simulink model "RoboBoatVU_2014_Athena"  (R2014a)
settings: Solver=FixedStepDiscrete  StartTime=0.0  StopTime=inf  FixedStep=.1  RelTol=1e-3
undefined symbols (not defined in the file): Com1, Com2, Com3, Com4, DiscIntNeverNeededParam, RGB24, standard, strel
libraries: visiontextngfix x25, dspmtrx3 x22, simulink x19, xpcseriallib x12, slrtlib x7, speedgoatlib_IO102 x6, dspstat3 x5, visionstatistics x3, dspindex x2, xpcvideousblib x2, xpcvideoutillib x2, visionmorphops x1
(part 4 of 4)

== matlab function RoboBoatVU_2014_Athena/Main FSM/Docking/Recognition/Recognition ==
  data: targetTemp input; bbox_out output; cruciform input; circle input; triangle input; whitePixCount input; threshold input; V_mask input; bbox_in input; returnRatioDiff output
function [bbox_out,returnRatioDiff] = recognition(targetTemp,cruciform,circle,triangle,...
    whitePixCount,threshold,V_mask,bbox_in)

% Written by Edward Zhu on 5/14/14

% Inputs
% tempID:       Number corresponding to one of the templates (cruciform: 1,
%               circle: 2, triangle: 3)
% cruciform:    19*19 template of cruciform
% circle:       19*19 template of circle
% triangle:     19*19 template of triangle
% whitePixCount:Number of white pixels in each of the templates
% V_mask:       V channel binary mask
% bbox_in:      Bounding boxes as found by blob analysis
% label:        Label matrix as found by blob analysis

% Outputs
% bbox_out:     Bounding box of matched symbol
% symFound:     Status of matching (found: 1, not found: 0)

% Define frame and template size
templates = zeros(19,19,3);
templates(:,:,1) = cruciform;
templates(:,:,2) = circle;
templates(:,:,3) = triangle;
templates = 2*(templates-0.5);

tempRows = size(templates,1);
tempCols = size(templates,2);
numBBox = size(bbox_in,1);

% Initialize scaled image and output bbox matrices
V_scaled = zeros(tempRows,tempCols);
bbox_out = uint32(zeros(numBBox,4));

returnRatioDiff = ones(numBBox,1);

for i = 1:numBBox
    if min(bbox_in(i,:)) > 0
        similarity = 0;
        rowScaleStep = floor(bbox_in(i,4) / tempRows);
        colScaleStep = floor(bbox_in(i,3) / tempCols);
        
        captureRow = bbox_in(i,2);
        for row = 1:tempRows
            captureCol = bbox_in(i,1);
            for col = 1:tempCols
                V_scaled(row,col) = V_mask(captureRow,captureCol);
                similarity = similarity + templates(row,col,targetTemp) * (V_mask(captureRow,captureCol)*(-1) + 1);
                captureCol = captureCol + colScaleStep;
            end
            captureRow = captureRow + rowScaleStep;
        end
        
        ratioDiff = abs(1 - single(similarity) / single(whitePixCount(targetTemp)));
        
        % Output valid bounding box
        if ratioDiff < threshold
            bbox_out(i,:) = bbox_in(i,:);
            returnRatioDiff(i) = ratioDiff;
        end
    end
end

== matlab function RoboBoatVU_2014_Athena/Main FSM/Docking/Video Annotation/x shift ==
  data: bbox_in input; bbox_out output
function bbox_out = x_shift(bbox_in)

bbox_out = [bbox_in(:,1) + 128, bbox_in(:,2),bbox_in(:,3),bbox_in(:,4)];

== matlab function RoboBoatVU_2014_Athena/Main FSM/Return to Start/GPS: Center/Approach/Desired Heading and Distance ==
  data: Distance output; DesiredGPS input; DesiredHeading output; GPSLat input; GPSLong input
function [Distance, DesiredHeading] = Approach(DesiredGPS, GPSLat, GPSLong)

%Written by Anderson Lebbad on July 22, 2013
%Last Edited:

%Orients the boat towards a target GPS point before approaching it.
%This is done to keep the approach angle minimal, so the approach
%algorithm does not circle the target and never reach it.

%Parse input GPS and convert angles to radians
CurLat = (floor(GPSLat/100)+mod(GPSLat,100)/60)*pi/180;
CurLong = (floor(GPSLong/100)+mod(GPSLong,100)/60)*pi/180;
DesLat = (floor(DesiredGPS(1)/100)+mod(DesiredGPS(1),100)/60)*pi/180;
DesLong = (floor(DesiredGPS(2)/100)+mod(DesiredGPS(2),100)/60)*pi/180;
%Difference between lats and longs
DiffLat = DesLat - CurLat;
DiffLong = DesLong - CurLong;
%Radius of the earth in meters
R = 6378137;

%Calculate distance using the great-circle distance formula
%Formula documented here:
%   http://www.movable-type.co.uk/scripts/latlong.html
a = sin(DiffLat/2)^2+sin(DiffLong/2)^2*cos(CurLat)*cos(DesLat);
c = 2*atan2(sqrt(a), sqrt(1-a));
Distance = R*c;

%Calculate initial bearing - formula documented here: 
%   http://www.movable-type.co.uk/scripts/latlong.html
y = sin(DiffLong)*cos(DesLat);
x = cos(CurLat)*sin(DesLat)-sin(CurLat)*cos(DesLat)*cos(DiffLong);
DesiredHeading = atan2(y, x);

%Make all angles positive
if DesiredHeading < 0
    DesiredHeading = DesiredHeading + 360;
end

== matlab function RoboBoatVU_2014_Athena/Main FSM/Return to Start/GPS: Center/Approach/Within Range ==
  data: GPSApproachDist input; Finished output; Distance input
function Finished = DistanceReached(GPSApproachDist, Distance)

%Written by Anderson Lebbad on July 22, 2013
%Last Edited:

%This function checks to see if the boat is within a set distance of the
%destination point to return a finished flag

%If the Distance is within the GPSApproachDist, the boat is close enough 
%to send a finished signal
if Distance < GPSApproachDist
    Finished = 1;
else
    Finished = 0;
end

== matlab function RoboBoatVU_2014_Athena/Main FSM/Return to Start/GPS: Center/GPS Enabler ==
  data: Finished input; GPSMode output; OrientEnable output; ApproachEnable output
function [GPSMode, OrientEnable, ApproachEnable] =...
    GPSEnable(Finished)

%Written by Anderson Lebbad on July 22, 2013
%Last Edited: July 27, 2013
%   Removed Termination Block

%This function enables GPS tasks. First the boat orients towards the
%target, then it approaches it.


%Parse Finished signal
OrientFinished = Finished(1);


%Initialize Enablers
OrientEnable = 0;
ApproachEnable = 0;


%Switches the enable signal based on which task is flagged as done.
if OrientFinished == 0
    OrientEnable = 1;
    GPSMode = 1;
else
    ApproachEnable = 1;
    GPSMode = 2;
end

== matlab function RoboBoatVU_2014_Athena/Main FSM/Return to Start/GPS: Center/Orient/Desired Heading ==
  data: DesiredGPS input; DesiredHeading output; GPSLat input; GPSLong input
function DesiredHeading = Orient(DesiredGPS, GPSLat, GPSLong)

%Written by Anderson Lebbad on July 22, 2013
%Last Edited:

%Orients the boat towards a target GPS point before approaching it.
%This is done to keep the approach angle minimal, so the approach
%algorithm does not circle the target and never reach it.

%Parse input GPS and convert angles to radians
CurLat = (floor(GPSLat/100)+mod(GPSLat,100)/60)*pi/180;
CurLong = (floor(GPSLong/100)+mod(GPSLong,100)/60)*pi/180;
DesLat = (floor(DesiredGPS(1)/100)+mod(DesiredGPS(1),100)/60)*pi/180;
DesLong = (floor(DesiredGPS(2)/100)+mod(DesiredGPS(2),100)/60)*pi/180;
%Difference between longs
DiffLong = DesLong - CurLong;

%Calculate initial bearing - formula documented here: 
%   http://www.movable-type.co.uk/scripts/latlong.html
y = sin(DiffLong)*cos(DesLat);
x = cos(CurLat)*sin(DesLat)-sin(CurLat)*cos(DesLat)*cos(DiffLong);
DesiredHeading = atan2(y, x)*180/pi;

%Make all angles positive
if DesiredHeading < 0
    DesiredHeading = DesiredHeading + 360;
end

== matlab function RoboBoatVU_2014_Athena/Main FSM/Acoustic Location/Mid Sample/MATLAB Function2 ==
  data: currentHeading input; desiredHeading output
function desiredHeading = holdHeading(currentHeading)
persistent heldHeading

if isempty(heldHeading)
    heldHeading = currentHeading;
end

desiredHeading = heldHeading;

== matlab function RoboBoatVU_2014_Athena/Main FSM/Acoustic Location/Left Sample/MATLAB Function2 ==
  data: currentHeading input; desiredHeading output
function desiredHeading = holdHeading(currentHeading)
persistent heldHeading

if isempty(heldHeading)
    heldHeading = currentHeading;
end

desiredHeading = heldHeading;

== matlab function RoboBoatVU_2014_Athena/Main FSM/Acoustic Location/Right Sample/MATLAB Function2 ==
  data: currentHeading input; desiredHeading output
function desiredHeading = holdHeading(currentHeading)
persistent heldHeading

if isempty(heldHeading)
    heldHeading = currentHeading;
end

desiredHeading = heldHeading;

== matlab function RoboBoatVU_2014_Athena/Main FSM/Return to Start/GPS: Center/Orient/Within Range ==
  data: DesiredHeading input; Finished output; Compass input
function Finished = OrientLocked(DesiredHeading, Compass)

%Written by Anderson Lebbad on July 22, 2013
%Last Edited:

%This function checks to see if the target heading has been reached and 
%sends a finished signal when it has.

HeadingDiff = DesiredHeading - Compass;

%Sets the range for the difference angle to be -180 to +180
if HeadingDiff > 180
    HeadingDiff = HeadingDiff - 360;
elseif HeadingDiff < -180
    HeadingDiff = HeadingDiff + 360;
end

%If the Heading is within 3 degrees, the angle is close enough to send a
%finished signal
if abs(HeadingDiff) < 3
    Finished = 1;
else
    Finished = 0;
end

== matlab function RoboBoatVU_2014_Athena/Main FSM/Obstacle Navigation/Silly Action Decider ==
  data: buoyColor input; desiredHeading output; currentHeading input; finished output
function [desiredHeading,finished]  = sillyActionDecider(buoyColor,currentHeading)
% Decides on which silly action for SeaCat to take based on the color of
% the buoy as read from the Pandaboard where red: 1, white: 2, green: 3
persistent heldHeading turnCount turn

desiredHeading = currentHeading;
finished = 0;

if buoyColor ~= 0
    
    if isempty(heldHeading) && isempty(turnCount) && isempty(turn)
        heldHeading = currentHeading;
        turnCount = 0;
        turn = 10;
    end

    switch buoyColor
        case 1
            desiredHeading = currentHeading + turn;
            if abs(desiredHeading-heldHeading) > 90
                desiredHeading = currentHeading;
                finished = 1;
            end
        case 2
            desiredHeading = currentHeading + turn;
            if abs(desiredHeading-heldHeading) > 90
                turn = -turn;
                turnCount = turnCount + 1;
                if turnCount > 2
                    desiredHeading = currentHeading;
                    finished = 1;
                end
            end
        case 3
            desiredHeading = currentHeading - turn;
            if abs(desiredHeading-heldHeading) > 90
                desiredHeading = currentHeading;
                finished = 1;
            end
    end
    
else
    desiredHeading = currentHeading;
    finished = 0;
end

== matlab function RoboBoatVU_2014_Athena/Main FSM/Color Sequence Detection/MATLAB Function ==
  data: testTimeout input; time input; finished output; colorLocateFin input; readReady output
function [finished,readReady] = arduinoReadEnable(testTimeout,time,colorLocateFin)

if colorLocateFin == 1
    readReady = 1;
else
    readReady = 0;
end

if time >= testTimeout
    finished = 1;
else
    finished = 0;
end

== matlab function RoboBoatVU_2014_Athena/Main FSM/Acoustic Location/MATLAB Function ==
  data: midSampleFin input; leftTurnFin input; leftSampleFin input; taskSelector output; midSampleEn output; rightTurnFin input; leftTurnEn output; leftSampleEn output; rightTurnEn output; rightSampleEn output
function [taskSelector,midSampleEn,leftTurnEn,leftSampleEn,...
    rightTurnEn,rightSampleEn] = hydrophoneTestEnabler(midSampleFin,...
    leftTurnFin,leftSampleFin,rightTurnFin)

midSampleEn = 0;
leftTurnEn = 0;
leftSampleEn = 0;
rightTurnEn = 0;
rightSampleEn = 0;


if midSampleFin == 0
    midSampleEn = 1;
    taskSelector = 1;
elseif leftTurnFin == 0
    leftTurnEn = 1;
    taskSelector = 2;
elseif leftSampleFin == 0
    leftSampleEn = 1;
    taskSelector = 3;
elseif rightTurnFin == 0
    rightTurnEn = 1;
    taskSelector = 4;
else
    rightSampleEn = 1;
    taskSelector = 5;
end

== matlab function RoboBoatVU_2014_Athena/Main FSM/Acoustic Location/Mid Sample/MATLAB Function ==
  data: testTimeout input; time input; finished output
function finished  = timeout(testTimeout,time)

if time >= testTimeout
    finished = 1;
else
    finished = 0;
end

== matlab function RoboBoatVU_2014_Athena/Main FSM/Acoustic Location/Left Sample/MATLAB Function ==
  data: testTimeout input; time input; finished output
function finished  = timeout(testTimeout,time)

if time >= testTimeout
    finished = 1;
else
    finished = 0;
end

== matlab function RoboBoatVU_2014_Athena/Main FSM/Acoustic Location/Right Sample/MATLAB Function ==
  data: testTimeout input; time input; finished output
function finished  = timeout(testTimeout,time)

if time >= testTimeout
    finished = 1;
else
    finished = 0;
end

== matlab function RoboBoatVU_2014_Athena/Main FSM/Acoustic Location/Left Turn/Left Turn ==
  data: desiredHeading output; currentHeading input; finished output
function [desiredHeading,finished]  = leftTurn(currentHeading)
% Decides on which silly action for SeaCat to take based on the color of
% the buoy as read from the Pandaboard where red: 1, white: 2, green: 3
persistent heldHeading turn lock counter

finished = 0;
desiredHeading = currentHeading;
turninc = 20;

if isempty(heldHeading) && isempty(turn) && isempty(lock) && isempty(counter)
    heldHeading = currentHeading;
    turn = 1;
    lock = 0;
    counter = 0;
end

if turn == 1 && lock == 0
    
desiredHeading = currentHeading - turninc;

    if abs(currentHeading-heldHeading) > 30
        heldHeading = currentHeading;
        turn = 0;
        lock = 1;
    end
    
finished = 0;

end

if turn == 0 && lock == 1
    
    desiredHeading = heldHeading;
    
    if abs(currentHeading - desiredHeading) <= 5
        counter = counter + 1;
    else
        counter = 0;
    end
    
    if counter < 10
        finished = 0;
    else
        finished = 1;
    end
    
end

== matlab function RoboBoatVU_2014_Athena/Main FSM/Acoustic Location/Right Turn/Right Turn ==
  data: desiredHeading output; currentHeading input; finished output
function [desiredHeading,finished]  = rightTurn(currentHeading)
% Decides on which silly action for SeaCat to take based on the color of
% the buoy as read from the Pandaboard where red: 1, white: 2, green: 3
persistent heldHeading turn lock counter

finished = 0;
desiredHeading = currentHeading;
turninc = 20;

if isempty(heldHeading) && isempty(turn) && isempty(lock) && isempty(counter)
    heldHeading = currentHeading;
    turn = 1;
    lock = 0;
    counter = 0;
end

if turn == 1 && lock == 0
    
desiredHeading = currentHeading + turninc;

    if abs(currentHeading-heldHeading) > 60
        heldHeading = currentHeading;
        turn = 0;
        lock = 1;
    end
    
finished = 0;

end

if turn == 0 && lock == 1
    
    desiredHeading = heldHeading;
    
    if abs(currentHeading - desiredHeading) <= 5
        counter = counter + 1;
    else
        counter = 0;
    end
    
    if counter < 10
        finished = 0;
    else
        finished = 1;
    end
    
end

== matlab function RoboBoatVU_2014_Athena/Sensors/Serial In/Decode Compass/Correct Heading Angle Magnetic to True North/Magnetic to True North Conversion ==
  data: HeadingM input; HeadingT output
function HeadingT = fcn(HeadingM)
% This block supports the Embedded MATLAB subset.
% See the help menu for details. 

HeadingT=HeadingM+180-12.3; %180 was added since compass was rotated when
                            %it was relocated.

if HeadingT>360
    HeadingT=HeadingT-360;
elseif HeadingT<0;
    HeadingT=HeadingT+360;
end

== matlab function RoboBoatVU_2014_Athena/Parameters/Task Selector/Message Composer ==
  data: taskStrInit input; taskStrAdj output
function taskStrAdj = composeMessage(taskStrInit)
%Written by Anderson Lebbad on August 9, 2013
%Last Edited: Edward Zhu on June 2, 2014

%This function adjusts the length of a vector to a set value by filling
%the remaining space with 0's. This is necessary for data store objects
%that have a fixed size for the memory allocation, but a variable length
%input.

%Length of message packet
strLength = 8;

%Size of text in message
taskStrLength = size(taskStrInit,1);

%Pad end of text with zeros
taskStrAdj = [taskStrInit' zeros(1,strLength-taskStrLength)];

== matlab function RoboBoatVU_2014_Athena/Parameters/Task Selector/Message Composer1 ==
  data: taskStrInit input; taskStrAdj output
function taskStrAdj = composeMessage(taskStrInit)
%Written by Anderson Lebbad on August 9, 2013
%Last Edited: Edward Zhu on June 2, 2014

%This function adjusts the length of a vector to a set value by filling
%the remaining space with 0's. This is necessary for data store objects
%that have a fixed size for the memory allocation, but a variable length
%input.

%Length of message packet
strLength = 8;

%Size of text in message
taskStrLength = size(taskStrInit,1);

%Pad end of text with zeros
taskStrAdj = [taskStrInit' zeros(1,strLength-taskStrLength)];

== matlab function RoboBoatVU_2014_Athena/Parameters/Task Selector/Message Composer4 ==
  data: taskStrInit input; taskStrAdj output
function taskStrAdj = composeMessage(taskStrInit)
%Written by Anderson Lebbad on August 9, 2013
%Last Edited: Edward Zhu on June 2, 2014

%This function adjusts the length of a vector to a set value by filling
%the remaining space with 0's. This is necessary for data store objects
%that have a fixed size for the memory allocation, but a variable length
%input.

%Length of message packet
strLength = 8;

%Size of text in message
taskStrLength = size(taskStrInit,1);

%Pad end of text with zeros
taskStrAdj = [taskStrInit' zeros(1,strLength-taskStrLength)];

== matlab function RoboBoatVU_2014_Athena/Parameters/Task Options/Fix length ==
  data: selection input; adjusted output
function adjusted = FixLength(selection)

%Written by Anderson Lebbad on August 9, 2013
%Last Edited:

%This function adjusts the length of a vector to a set value by filling
%the remaining space with 0's. This is necessary for data store objects
%that have a fixed size for the memory allocation, but a variable length
%input.


%Required length
set = 8;


%input length
current = length(selection);


%Pad with zeros
adjusted = [selection' zeros(1, set-current)];
